simulink model "CP_ContrSys_NLin_n9464263"  (R2020a)
settings: Solver=VariableStepAuto  StartTime=0.0  StopTime=10.0  RelTol=1e-3
values from neighbouring files (symbols this model uses):
  K = place(A, B, [-3, -4, -5, -6])    [nonlinear_dynamics.m]
  x0 = [0.2 20*pi/180 0 0]'    [CP_ContrSys_a_MainFile_n9464263.m]    (also in CP_ContrSys_b_MainFile_n9464263.m = [0.2 200*pi/180 0 0]'; nonlinear_dynamics.m = [0 0 0 0]')
settings Model: Creator=cal  LastModifiedBy=cal

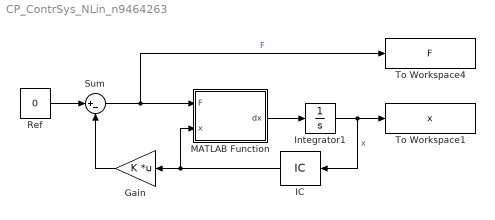
== system CP_ContrSys_NLin_n9464263 ==
  Gain : Gain  Gain=K  Multiplication=Matrix(K*u)
  IC : InitialCondition  Value=x0
  Integrator1 : Integrator
  MATLAB Function : MATLAB Function  TreatAsAtomicUnit=on
  Ref : Constant  Value=0
  Sum : Sum  Inputs=|+-
  To Workspace1 : ToWorkspace  VariableName=x  SampleTime=-1
  To Workspace4 : ToWorkspace  VariableName=F  SampleTime=-1
  wires:
  Integrator1/1 -> IC/1, To Workspace1/1  "x"
  MATLAB Function/1(dx) -> Integrator1/1
  Sum/1 -> To Workspace4/1, MATLAB Function/1(F)  "F"
  IC/1 -> Gain/1, MATLAB Function/2(x)
  Ref/1 -> Sum/1
  Gain/1 -> Sum/2

== matlab function CP_ContrSys_NLin_n9464263/MATLAB Function ==
  data: F input; dx output; x input
function dx = fcn(F, x)
dx = zeros(size(x));
dx = nonlinear_dynamics_plant(F, x);
